simulink model "Experiment_2_cs"  (Simulink 8.4)
settings: Solver=ode5  SolverMode=SingleTasking  StartTime=0.0  StopTime=inf  FixedStep=1/100  RelTol=1e-3
PreLoadFcn:
  | mbxruntime.callbacks.PreLoadFcn(bdroot);
PostLoadFcn:
  | mbxruntime.callbacks.PostLoadFcn(bdroot);
InitFcn:
  | mbxruntime.callbacks.InitFcn(bdroot);
StartFcn:
  | mbxruntime.callbacks.StartFcn(bdroot);
StopFcn:
  | mbxruntime.callbacks.StopFcn(bdroot);
undefined symbols (not defined in the file or in its folder): dfreq, gray, InitImageOutputDir, Rec, SDTV, strel, warningInitialVelocity, x0
libraries: simulink x43, PreScanSimulinkLibrary x19, visiontextngfix x15, simulink_extras x11, visionconversions x3, PreScanUsefulBlocks x3, visionsinks x2, visionstatistics x1, visionmorphops x1, visionanalysis x1
(part 5 of 8)

== system Experiment_2_cs/Audi_A8_1/ENABLED/Trajectories/TrajCoGOffset ==
  State In : Inport
  Add : Sum  Inputs=+-+
  Add1 : Sum
  ApplyRotation : PreScanSimulinkLibrary/ApplyRotation
  ApplyRotation1 : PreScanSimulinkLibrary/ApplyRotation
  CoG Offset : Constant  Value=[0 0 CoGOffsetZ]
  Degrees to Radians : simulink_extras/Transformations/Degrees to Radians
  Demux1 : Demux  Outputs=[3 3 3]
  Mux : Mux  Inputs=[3 3 3]
  Orientation : Constant  Value=[InitRoll InitPitch 0]
  State Out : Outport
  wires:
  State In/1 -> Demux1/1
  Demux1/1 -> Add/1
  Add/1 -> Mux/1
  Demux1/3 -> Mux/3, Add1/2
  Mux/1 -> State Out/1
  Demux1/2 -> Mux/2
  Orientation/1 -> Degrees to Radians/1
  ApplyRotation/1 -> Add/3
  ApplyRotation1/1 -> Add/2
  Add1/1 -> ApplyRotation/2
  CoG Offset/1 -> ApplyRotation1/1, ApplyRotation/1
  Degrees to Radians/1 -> Add1/1, ApplyRotation1/2

== system Experiment_2_cs/Audi_A8_1/ENABLED/Trajectories/Trajectory_2 ==
  From Workspace : FromWorkspace  VariableName=trajectory  SampleTime=TimeStep  OutputAfterFinalValue=Holding final value
  From Workspace1 : FromWorkspace  VariableName=trajectory  SampleTime=TimeStep  OutputAfterFinalValue=Setting to zero
  Mux : Mux  Inputs=2
  Selector1 : Selector  InputPortWidth=24  Indices=[7:18]
  Selector9 : Selector  InputPortWidth=24  Indices=[1:6]
  trajectory : Outport
  wires:
  From Workspace/1 -> Selector9/1
  From Workspace1/1 -> Selector1/1
  Mux/1 -> trajectory/1
  Selector9/1 -> Mux/1
  Selector1/1 -> Mux/2

== system Experiment_2_cs/Audi_A8_1/ENABLED/V2X_210_Generic_Filter/Filter ==
  In : Inport
  Filter : MATLAB Function  TreatAsAtomicUnit=on
  Zero : Constant  Value=0  OutDataTypeStr=Bus: PRESCAN_V2X_USER_GENERIC_MESSAGE
  Out : Outport
  wires:
  Zero/1 -> Filter/2(z)
  Filter/1(y) -> Out/1
  In/1 -> Filter/1(u)

== system Experiment_2_cs/BMW_Z3_1/ENABLED/SELF_Demux/compas converter ==
  rotz [rad] : Inport
  cart2compas : Subsystem
  rad2deg : Gain  Gain=180/pi
  heading [deg] : Outport
  wires:
  rad2deg/1 -> cart2compas/1(Angle [deg])
  rotz [rad]/1 -> rad2deg/1
  cart2compas/1(heading [deg]) -> heading [deg]/1

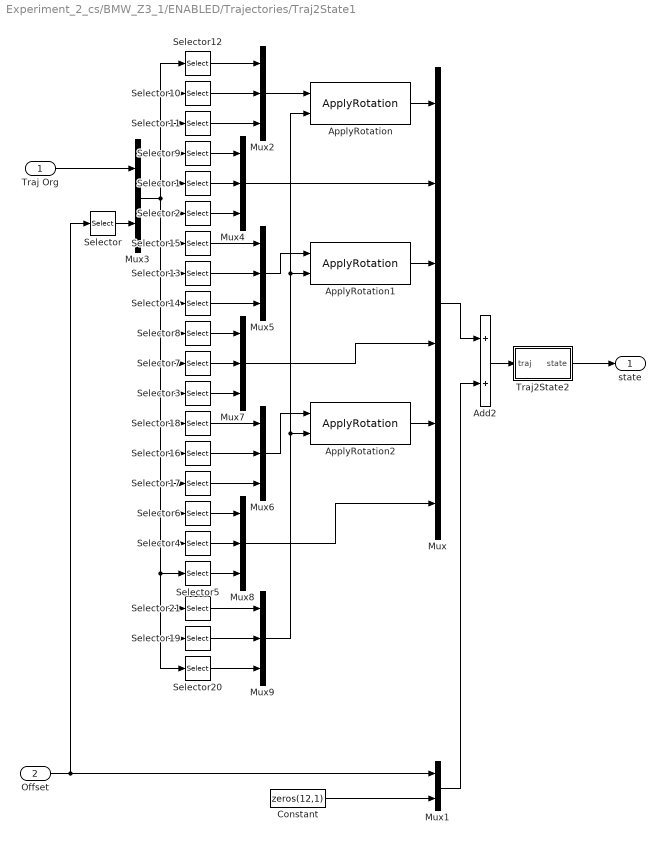
== system Experiment_2_cs/BMW_Z3_1/ENABLED/Trajectories/Traj2State1 ==
  Traj Org : Inport
  Offset : Inport  Port=2
  Add2 : Sum
  ApplyRotation : PreScanSimulinkLibrary/ApplyRotation
  ApplyRotation1 : PreScanSimulinkLibrary/ApplyRotation
  ApplyRotation2 : PreScanSimulinkLibrary/ApplyRotation
  Constant : Constant  Value=zeros(12,1)
  Mux : Mux  Inputs=6
  Mux1 : Mux  Inputs=2
  Mux{2,4..9} (7 alike) : Mux  Inputs=3
  Mux3 : Mux  Inputs=2
  Selector : Selector  InputPortWidth=6  Indices=[4 5 6]
  Selector1 : Selector  InputPortWidth=21  Indices=[5]
  Selector10 : Selector  InputPortWidth=21  Indices=[2]
  Selector11 : Selector  InputPortWidth=21  Indices=[3]
  Selector12 : Selector  InputPortWidth=21  Indices=[1]
  Selector13 : Selector  InputPortWidth=21  Indices=[8]
  Selector14 : Selector  InputPortWidth=21  Indices=[9]
  Selector15 : Selector  InputPortWidth=21  Indices=[7]
  Selector16 : Selector  InputPortWidth=21  Indices=[14]
  Selector17 : Selector  InputPortWidth=21  Indices=[15]
  Selector18 : Selector  InputPortWidth=21  Indices=[13]
  Selector19 : Selector  InputPortWidth=21  Indices=[20]
  Selector2 : Selector  InputPortWidth=21  Indices=[6]
  Selector20 : Selector  InputPortWidth=21  Indices=[21]
  Selector21 : Selector  InputPortWidth=21  Indices=[19]
  Selector3 : Selector  InputPortWidth=21  Indices=[12]
  Selector4 : Selector  InputPortWidth=21  Indices=[17]
  Selector5 : Selector  InputPortWidth=21  Indices=[18]
  Selector6 : Selector  InputPortWidth=21  Indices=[16]
  Selector7 : Selector  InputPortWidth=21  Indices=[11]
  Selector8 : Selector  InputPortWidth=21  Indices=[10]
  Selector9 : Selector  InputPortWidth=21  Indices=[4]
  Traj2State2 : Subsystem
  state : Outport
  wires:
  Mux9/1 -> ApplyRotation2/2, ApplyRotation1/2, ApplyRotation/2
  Selector20/1 -> Mux9/3
  Selector19/1 -> Mux9/2
  Selector21/1 -> Mux9/1
  Selector5/1 -> Mux8/3
  Selector4/1 -> Mux8/2
  Selector6/1 -> Mux8/1
  Mux8/1 -> Mux/6
  Mux6/1 -> ApplyRotation2/1
  Mux7/1 -> Mux/4
  ApplyRotation2/1 -> Mux/5
  Selector3/1 -> Mux7/3
  Selector7/1 -> Mux7/2
  Selector8/1 -> Mux7/1
  Mux4/1 -> Mux/2
  Mux5/1 -> ApplyRotation1/1
  ApplyRotation1/1 -> Mux/3
  Mux2/1 -> ApplyRotation/1
  ApplyRotation/1 -> Mux/1
  Selector2/1 -> Mux4/3
  Selector1/1 -> Mux4/2
  Selector9/1 -> Mux4/1
  Selector17/1 -> Mux6/3
  Selector16/1 -> Mux6/2
  Selector18/1 -> Mux6/1
  Selector14/1 -> Mux5/3
  Selector13/1 -> Mux5/2
  Selector15/1 -> Mux5/1
  Selector11/1 -> Mux2/3
  Selector10/1 -> Mux2/2
  Selector12/1 -> Mux2/1
  Mux3/1 -> Selector8/1, Selector7/1, Selector3/1, Selector18/1, Selector16/1, Selector17/1, Selector6/1, Selector20/1, Selector19/1, Selector21/1, Selector5/1, Selector4/1, Selector14/1, Selector13/1, Selector15/1, Selector2/1, Selector1/1, Selector9/1, Selector12/1, Selector10/1, Selector11/1
  Mux1/1 -> Add2/2
  Constant/1 -> Mux1/2
  Add2/1 -> Traj2State2/1(traj)
  Selector/1 -> Mux3/2
  Traj Org/1 -> Mux3/1
  Offset/1 -> Mux1/1, Selector/1
  Mux/1 -> Add2/1
  Traj2State2/1(state) -> state/1

== system Experiment_2_cs/BMW_Z3_1/ENABLED/Trajectories/TrajCoGOffset ==
  State In : Inport
  Add : Sum  Inputs=+-+
  Add1 : Sum
  ApplyRotation : PreScanSimulinkLibrary/ApplyRotation
  ApplyRotation1 : PreScanSimulinkLibrary/ApplyRotation
  CoG Offset : Constant  Value=[0 0 CoGOffsetZ]
  Degrees to Radians : simulink_extras/Transformations/Degrees to Radians
  Demux1 : Demux  Outputs=[3 3 3]
  Mux : Mux  Inputs=[3 3 3]
  Orientation : Constant  Value=[InitRoll InitPitch 0]
  State Out : Outport
  wires:
  State In/1 -> Demux1/1
  Demux1/1 -> Add/1
  Add/1 -> Mux/1
  Demux1/3 -> Mux/3, Add1/2
  Mux/1 -> State Out/1
  Demux1/2 -> Mux/2
  Orientation/1 -> Degrees to Radians/1
  ApplyRotation/1 -> Add/3
  ApplyRotation1/1 -> Add/2
  Add1/1 -> ApplyRotation/2
  CoG Offset/1 -> ApplyRotation1/1, ApplyRotation/1
  Degrees to Radians/1 -> Add1/1, ApplyRotation1/2

== system Experiment_2_cs/BMW_Z3_1/ENABLED/Trajectories/Trajectory_3 ==
  From Workspace : FromWorkspace  VariableName=trajectory  SampleTime=TimeStep  OutputAfterFinalValue=Holding final value
  From Workspace1 : FromWorkspace  VariableName=trajectory  SampleTime=TimeStep  OutputAfterFinalValue=Setting to zero
  Mux : Mux  Inputs=2
  Selector1 : Selector  InputPortWidth=24  Indices=[7:18]
  Selector9 : Selector  InputPortWidth=24  Indices=[1:6]
  trajectory : Outport
  wires:
  From Workspace/1 -> Selector9/1
  From Workspace1/1 -> Selector1/1
  Mux/1 -> trajectory/1
  Selector9/1 -> Mux/1
  Selector1/1 -> Mux/2

== system Experiment_2_cs/BMW_Z3_1/ENABLED/V2X_211_Generic_Filter/Filter ==
  In : Inport
  Filter : MATLAB Function  TreatAsAtomicUnit=on
  Zero : Constant  Value=0  OutDataTypeStr=Bus: PRESCAN_V2X_USER_GENERIC_MESSAGE
  Out : Outport
  wires:
  Zero/1 -> Filter/2(z)
  Filter/1(y) -> Out/1
  In/1 -> Filter/1(u)

== system Experiment_2_cs/CollisionDetection/DISABLED/GND1/GND_DATA ==
  GND_ObjectID1 : Constant  Value=uint32(0)
  GND_ObjectID2 : Constant  Value=uint32(0)
  buscreator : BusCreator  Inputs=2  OutDataTypeStr=Bus: PRESCAN_COLLISIONDETECTION_DATA  NonVirtualBus=on
  bus : Outport  OutDataTypeStr=Bus: PRESCAN_COLLISIONDETECTION_DATA
  wires:
  GND_ObjectID1/1 -> buscreator/1  "ObjectID1"
  GND_ObjectID2/1 -> buscreator/2  "ObjectID2"
  buscreator/1 -> bus/1

== system Experiment_2_cs/CollisionDetection/DISABLED/GND1/GND_HEADER ==
  GND_valid : Constant  Value=boolean(0)
  buscreator : BusCreator  Inputs=1  OutDataTypeStr=Bus: PRESCAN_HEADER  NonVirtualBus=on
  bus : Outport  OutDataTypeStr=Bus: PRESCAN_HEADER
  wires:
  GND_valid/1 -> buscreator/1  "valid"
  buscreator/1 -> bus/1

== system Experiment_2_cs/Male_RegularAni_1/ENABLED/Animation/animation mode ==
  vel : Inport
  Data Type Conversion : DataTypeConversion  OutDataTypeStr=double
  Fcn : Fcn  Expr=sqrt(u(1)^2+u(2)^2+u(3)^2)
  Running : simulink/Logic and Bit Operations/Compare To Constant  relop=>=  const=MWS  OutDataTypeStr=uint8  ZeroCross=off
  Sum : Sum  Inputs=|++
  Walking : simulink/Logic and Bit Operations/Compare To Zero  relop=~=  OutDataTypeStr=uint8  ZeroCross=off
  mode : Outport
  wires:
  vel/1 -> Fcn/1
  Sum/1 -> Data Type Conversion/1
  Walking/1 -> Sum/1
  Running/1 -> Sum/2
  Fcn/1 -> Walking/1, Running/1
  Data Type Conversion/1 -> mode/1

== system Experiment_2_cs/Male_RegularAni_1/ENABLED/Animation/elapsed track ==
  vel : Inport
  Discrete-Time Integrator : DiscreteIntegrator  SampleTime=-1
  Fcn : Fcn  Expr=sqrt(u(1)^2 + u(2)^2 + u(3)^2)
  s : Outport
  wires:
  Fcn/1 -> Discrete-Time Integrator/1
  vel/1 -> Fcn/1
  Discrete-Time Integrator/1 -> s/1

== system Experiment_2_cs/Male_RegularAni_1/ENABLED/SELF_Demux/compas converter ==
  rotz [rad] : Inport
  cart2compas : Subsystem
  rad2deg : Gain  Gain=180/pi
  heading [deg] : Outport
  wires:
  rad2deg/1 -> cart2compas/1(Angle [deg])
  rotz [rad]/1 -> rad2deg/1
  cart2compas/1(heading [deg]) -> heading [deg]/1

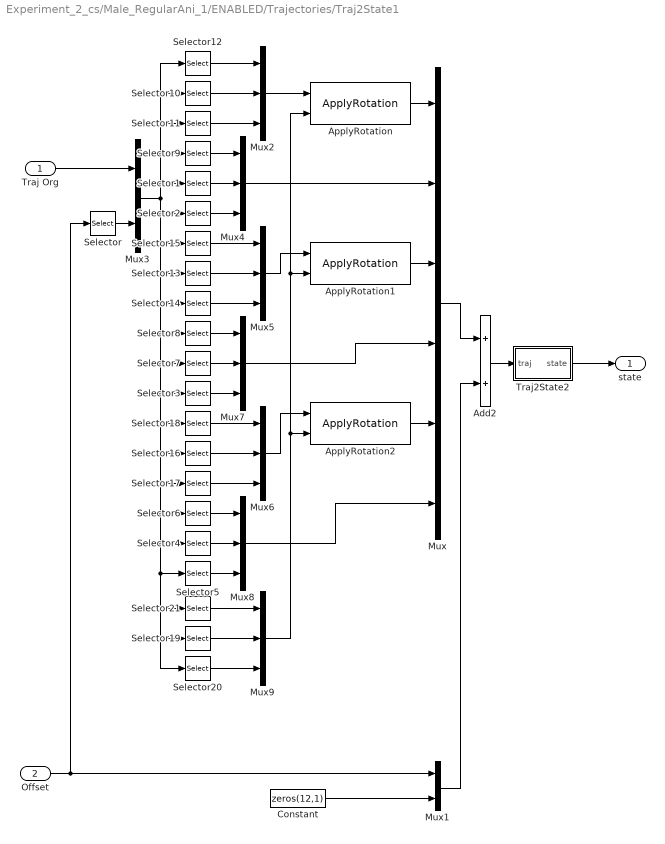
== system Experiment_2_cs/Male_RegularAni_1/ENABLED/Trajectories/Traj2State1 ==
  Traj Org : Inport
  Offset : Inport  Port=2
  Add2 : Sum
  ApplyRotation : PreScanSimulinkLibrary/ApplyRotation
  ApplyRotation1 : PreScanSimulinkLibrary/ApplyRotation
  ApplyRotation2 : PreScanSimulinkLibrary/ApplyRotation
  Constant : Constant  Value=zeros(12,1)
  Mux : Mux  Inputs=6
  Mux1 : Mux  Inputs=2
  Mux{2,4..9} (7 alike) : Mux  Inputs=3
  Mux3 : Mux  Inputs=2
  Selector : Selector  InputPortWidth=6  Indices=[4 5 6]
  Selector1 : Selector  InputPortWidth=21  Indices=[5]
  Selector10 : Selector  InputPortWidth=21  Indices=[2]
  Selector11 : Selector  InputPortWidth=21  Indices=[3]
  Selector12 : Selector  InputPortWidth=21  Indices=[1]
  Selector13 : Selector  InputPortWidth=21  Indices=[8]
  Selector14 : Selector  InputPortWidth=21  Indices=[9]
  Selector15 : Selector  InputPortWidth=21  Indices=[7]
  Selector16 : Selector  InputPortWidth=21  Indices=[14]
  Selector17 : Selector  InputPortWidth=21  Indices=[15]
  Selector18 : Selector  InputPortWidth=21  Indices=[13]
  Selector19 : Selector  InputPortWidth=21  Indices=[20]
  Selector2 : Selector  InputPortWidth=21  Indices=[6]
  Selector20 : Selector  InputPortWidth=21  Indices=[21]
  Selector21 : Selector  InputPortWidth=21  Indices=[19]
  Selector3 : Selector  InputPortWidth=21  Indices=[12]
  Selector4 : Selector  InputPortWidth=21  Indices=[17]
  Selector5 : Selector  InputPortWidth=21  Indices=[18]
  Selector6 : Selector  InputPortWidth=21  Indices=[16]
  Selector7 : Selector  InputPortWidth=21  Indices=[11]
  Selector8 : Selector  InputPortWidth=21  Indices=[10]
  Selector9 : Selector  InputPortWidth=21  Indices=[4]
  Traj2State2 : Subsystem
  state : Outport
  wires:
  Mux9/1 -> ApplyRotation2/2, ApplyRotation1/2, ApplyRotation/2
  Selector20/1 -> Mux9/3
  Selector19/1 -> Mux9/2
  Selector21/1 -> Mux9/1
  Selector5/1 -> Mux8/3
  Selector4/1 -> Mux8/2
  Selector6/1 -> Mux8/1
  Mux8/1 -> Mux/6
  Mux6/1 -> ApplyRotation2/1
  Mux7/1 -> Mux/4
  ApplyRotation2/1 -> Mux/5
  Selector3/1 -> Mux7/3
  Selector7/1 -> Mux7/2
  Selector8/1 -> Mux7/1
  Mux4/1 -> Mux/2
  Mux5/1 -> ApplyRotation1/1
  ApplyRotation1/1 -> Mux/3
  Mux2/1 -> ApplyRotation/1
  ApplyRotation/1 -> Mux/1
  Selector2/1 -> Mux4/3
  Selector1/1 -> Mux4/2
  Selector9/1 -> Mux4/1
  Selector17/1 -> Mux6/3
  Selector16/1 -> Mux6/2
  Selector18/1 -> Mux6/1
  Selector14/1 -> Mux5/3
  Selector13/1 -> Mux5/2
  Selector15/1 -> Mux5/1
  Selector11/1 -> Mux2/3
  Selector10/1 -> Mux2/2
  Selector12/1 -> Mux2/1
  Mux3/1 -> Selector8/1, Selector7/1, Selector3/1, Selector18/1, Selector16/1, Selector17/1, Selector6/1, Selector20/1, Selector19/1, Selector21/1, Selector5/1, Selector4/1, Selector14/1, Selector13/1, Selector15/1, Selector2/1, Selector1/1, Selector9/1, Selector12/1, Selector10/1, Selector11/1
  Mux1/1 -> Add2/2
  Constant/1 -> Mux1/2
  Add2/1 -> Traj2State2/1(traj)
  Selector/1 -> Mux3/2
  Traj Org/1 -> Mux3/1
  Offset/1 -> Mux1/1, Selector/1
  Mux/1 -> Add2/1
  Traj2State2/1(state) -> state/1

== system Experiment_2_cs/Male_RegularAni_1/ENABLED/Trajectories/TrajCoGOffset ==
  State In : Inport
  Add : Sum  Inputs=+-+
  Add1 : Sum
  ApplyRotation : PreScanSimulinkLibrary/ApplyRotation
  ApplyRotation1 : PreScanSimulinkLibrary/ApplyRotation
  CoG Offset : Constant  Value=[0 0 CoGOffsetZ]
  Degrees to Radians : simulink_extras/Transformations/Degrees to Radians
  Demux1 : Demux  Outputs=[3 3 3]
  Mux : Mux  Inputs=[3 3 3]
  Orientation : Constant  Value=[InitRoll InitPitch 0]
  State Out : Outport
  wires:
  State In/1 -> Demux1/1
  Demux1/1 -> Add/1
  Add/1 -> Mux/1
  Demux1/3 -> Mux/3, Add1/2
  Mux/1 -> State Out/1
  Demux1/2 -> Mux/2
  Orientation/1 -> Degrees to Radians/1
  ApplyRotation/1 -> Add/3
  ApplyRotation1/1 -> Add/2
  Add1/1 -> ApplyRotation/2
  CoG Offset/1 -> ApplyRotation1/1, ApplyRotation/1
  Degrees to Radians/1 -> Add1/1, ApplyRotation1/2

== system Experiment_2_cs/Male_RegularAni_1/ENABLED/Trajectories/Trajectory_1 ==
  From Workspace : FromWorkspace  VariableName=trajectory  SampleTime=TimeStep  OutputAfterFinalValue=Holding final value
  From Workspace1 : FromWorkspace  VariableName=trajectory  SampleTime=TimeStep  OutputAfterFinalValue=Setting to zero
  Mux : Mux  Inputs=2
  Selector1 : Selector  InputPortWidth=24  Indices=[7:18]
  Selector9 : Selector  InputPortWidth=24  Indices=[1:6]
  trajectory : Outport
  wires:
  From Workspace/1 -> Selector9/1
  From Workspace1/1 -> Selector1/1
  Mux/1 -> trajectory/1
  Selector9/1 -> Mux/1
  Selector1/1 -> Mux/2

== system Experiment_2_cs/TIS_1/DISABLED/GND1/GND_DATA ==
  GND_ActiveBeamID : Constant  Value=uint32(0)
  GND_Alpha : Constant  Value=0
  GND_Beta : Constant  Value=0
  GND_DopplerVelocity : Constant  Value=0
  GND_DopplerVelocityRotationX : Constant  Value=0
  GND_DopplerVelocityRotationY : Constant  Value=0
  GND_DopplerVelocityRotationZ : Constant  Value=0
  GND_DopplerVelocityTranslationX : Constant  Value=0
  GND_DopplerVelocityTranslationY : Constant  Value=0
  GND_DopplerVelocityTranslationZ : Constant  Value=0
  GND_EnergyLoss : Constant  Value=0
  GND_Phi : Constant  Value=0
  GND_Range : Constant  Value=0
  GND_TargetID : Constant  Value=uint32(0)
  GND_TargetTypeID : Constant  Value=uint32(0)
  GND_Theta : Constant  Value=0
  buscreator : BusCreator  Inputs=16  OutDataTypeStr=Bus: PRESCAN_SCANNERSENSOR_DATA  NonVirtualBus=on
  bus : Outport  OutDataTypeStr=Bus: PRESCAN_SCANNERSENSOR_DATA
  wires:
  GND_ActiveBeamID/1 -> buscreator/1  "ActiveBeamID"
  GND_Range/1 -> buscreator/2  "Range"
  GND_DopplerVelocity/1 -> buscreator/3  "DopplerVelocity"
  GND_Theta/1 -> buscreator/4  "Theta"
  GND_Phi/1 -> buscreator/5  "Phi"
  GND_TargetID/1 -> buscreator/6  "TargetID"
  GND_TargetTypeID/1 -> buscreator/7  "TargetTypeID"
  GND_EnergyLoss/1 -> buscreator/8  "EnergyLoss"
  GND_Alpha/1 -> buscreator/9  "Alpha"
  GND_Beta/1 -> buscreator/10  "Beta"
  GND_DopplerVelocityTranslationX/1 -> buscreator/11  "DopplerVelocityTranslationX"
  GND_DopplerVelocityTranslationY/1 -> buscreator/12  "DopplerVelocityTranslationY"
  GND_DopplerVelocityTranslationZ/1 -> buscreator/13  "DopplerVelocityTranslationZ"
  GND_DopplerVelocityRotationX/1 -> buscreator/14  "DopplerVelocityRotationX"
  GND_DopplerVelocityRotationY/1 -> buscreator/15  "DopplerVelocityRotationY"
  GND_DopplerVelocityRotationZ/1 -> buscreator/16  "DopplerVelocityRotationZ"
  buscreator/1 -> bus/1

== system Experiment_2_cs/TIS_1/DISABLED/GND1/GND_HEADER ==
  GND_valid : Constant  Value=boolean(0)
  buscreator : BusCreator  Inputs=1  OutDataTypeStr=Bus: PRESCAN_HEADER  NonVirtualBus=on
  bus : Outport  OutDataTypeStr=Bus: PRESCAN_HEADER
  wires:
  GND_valid/1 -> buscreator/1  "valid"
  buscreator/1 -> bus/1

== system Experiment_2_cs/TIS_2/DISABLED/GND1/GND_DATA ==
  GND_ActiveBeamID : Constant  Value=uint32(0)
  GND_Alpha : Constant  Value=0
  GND_Beta : Constant  Value=0
  GND_DopplerVelocity : Constant  Value=0
  GND_DopplerVelocityRotationX : Constant  Value=0
  GND_DopplerVelocityRotationY : Constant  Value=0
  GND_DopplerVelocityRotationZ : Constant  Value=0
  GND_DopplerVelocityTranslationX : Constant  Value=0
  GND_DopplerVelocityTranslationY : Constant  Value=0
  GND_DopplerVelocityTranslationZ : Constant  Value=0
  GND_EnergyLoss : Constant  Value=0
  GND_Phi : Constant  Value=0
  GND_Range : Constant  Value=0
  GND_TargetID : Constant  Value=uint32(0)
  GND_TargetTypeID : Constant  Value=uint32(0)
  GND_Theta : Constant  Value=0
  buscreator : BusCreator  Inputs=16  OutDataTypeStr=Bus: PRESCAN_SCANNERSENSOR_DATA  NonVirtualBus=on
  bus : Outport  OutDataTypeStr=Bus: PRESCAN_SCANNERSENSOR_DATA
  wires:
  GND_ActiveBeamID/1 -> buscreator/1  "ActiveBeamID"
  GND_Range/1 -> buscreator/2  "Range"
  GND_DopplerVelocity/1 -> buscreator/3  "DopplerVelocity"
  GND_Theta/1 -> buscreator/4  "Theta"
  GND_Phi/1 -> buscreator/5  "Phi"
  GND_TargetID/1 -> buscreator/6  "TargetID"
  GND_TargetTypeID/1 -> buscreator/7  "TargetTypeID"
  GND_EnergyLoss/1 -> buscreator/8  "EnergyLoss"
  GND_Alpha/1 -> buscreator/9  "Alpha"
  GND_Beta/1 -> buscreator/10  "Beta"
  GND_DopplerVelocityTranslationX/1 -> buscreator/11  "DopplerVelocityTranslationX"
  GND_DopplerVelocityTranslationY/1 -> buscreator/12  "DopplerVelocityTranslationY"
  GND_DopplerVelocityTranslationZ/1 -> buscreator/13  "DopplerVelocityTranslationZ"
  GND_DopplerVelocityRotationX/1 -> buscreator/14  "DopplerVelocityRotationX"
  GND_DopplerVelocityRotationY/1 -> buscreator/15  "DopplerVelocityRotationY"
  GND_DopplerVelocityRotationZ/1 -> buscreator/16  "DopplerVelocityRotationZ"
  buscreator/1 -> bus/1

== system Experiment_2_cs/TIS_2/DISABLED/GND1/GND_HEADER ==
  GND_valid : Constant  Value=boolean(0)
  buscreator : BusCreator  Inputs=1  OutDataTypeStr=Bus: PRESCAN_HEADER  NonVirtualBus=on
  bus : Outport  OutDataTypeStr=Bus: PRESCAN_HEADER
  wires:
  GND_valid/1 -> buscreator/1  "valid"
  buscreator/1 -> bus/1

== system Experiment_2_cs/Audi_A8_1/ENABLED/Dynamics_Simple/Chassis/Bicycle_model_[XYZ] ==
  DeltaWheel_[rad] : Inport
  zFront_[m]_dzFront_[ms-1] : Inport  Port=2  PortDimensions=2
  zRear_[m]_dzRear_[ms-1] : Inport  Port=3  PortDimensions=2
  BrakePressure_[bar] : Inport  Port=4
  DriveTorque_[Nm] : Inport  Port=5
  v0_[ms-1] : Inport  Port=6
  |vx|_[ms-1] : Inport  Port=7
  Fy_rear_[N] : Inport  Port=8
  Fy_front_[N] : Inport  Port=9
  Demux : Demux  Outputs=2
  Demux1 : Demux  Outputs=2
  Fyi --> Fy / Mz : Subsystem
  X_Motion : Subsystem
  Y & Yaw_Motion : Subsystem
  "Z, Pitch_Motion & Roll_Motion" : Subsystem
  |vx|_[ms-1]1 : Outport
  vy_[ms-1] : Outport  Port=2
  vz_[ms-1] : Outport  Port=3
  RollAngle_[rad] : Outport  Port=4
  RollRate_[rads-1] : Outport  Port=5
  YawAngle_[rads-1] : Outport  Port=6
  Vx_[ms-1] : Outport  Port=7
  PitchAngle_[rad] : Outport  Port=8
  YawAngle_[rad] : Outport  Port=9
  ax_[ms-2] : Outport  Port=10
  ay_[ms-2] : Outport  Port=11
  wires:
  Fyi --> Fy / Mz/1(Fy_[N]) -> Y & Yaw_Motion/2(Fy_[N])  "Fy_[N]"
  Fyi --> Fy / Mz/2(Mz_[Nm]) -> Y & Yaw_Motion/3(Mz_[Nm])  "Mz_[Nm]"
  Y & Yaw_Motion/1(|vx|_[ms-1]1) -> |vx|_[ms-1]1/1  "|vx|_[ms-1]"
  Y & Yaw_Motion/2(vy_[ms-1]) -> vy_[ms-1]/1  "vy_[ms-1]"
  Y & Yaw_Motion/5(YawAngle_[rad]) -> YawAngle_[rad]/1  "YawAngle_[rad]"
  v0_[ms-1]/1 -> X_Motion/3(v0_[ms-1])  "v0_[ms-1]"
  BrakePressure_[bar]/1 -> X_Motion/2(BrakePressure_[bar])  "BrakePressure_[bar]"
  DriveTorque_[Nm]/1 -> X_Motion/1(DriveTorque_[Nm])  "DriveTorque_[Nm]"
  X_Motion/2(ax_[ms-2]) -> ax_[ms-2]/1, [ax]  "ax_[ms-2]"
  X_Motion/1(vx_[ms-1]) -> Vx_[ms-1]/1, [vx]  "vx_[ms-1]"
  [ax] -> "Z, Pitch_Motion & Roll_Motion"/3(ax)
  Demux/1 -> "Z, Pitch_Motion & Roll_Motion"/5(zFront_[m])
  Demux/2 -> "Z, Pitch_Motion & Roll_Motion"/6(dzFront_[ms-1])
  Demux1/1 -> "Z, Pitch_Motion & Roll_Motion"/7(zRear_[m])
  Demux1/2 -> "Z, Pitch_Motion & Roll_Motion"/8(dzRear_[ms-1])
  zRear_[m]_dzRear_[ms-1]/1 -> Demux1/1
  zFront_[m]_dzFront_[ms-1]/1 -> Demux/1
  "Z, Pitch_Motion & Roll_Motion"/2(vz_[ms-1]) -> vz_[ms-1]/1  "vz_[ms-1]"
  DeltaWheel_[rad]/1 -> Fyi --> Fy / Mz/1(DeltaWheel_[rad])
  Fy_front_[N]/1 -> Fyi --> Fy / Mz/2(Fy_f_[N])
  Fy_rear_[N]/1 -> Fyi --> Fy / Mz/3(Fy_r_[N])
  |vx|_[ms-1]/1 -> Y & Yaw_Motion/1(|vx|_[ms-1])
  Y & Yaw_Motion/3(ay_[ms-2]) -> [ay], ay_[ms-2]/1  "ay_[ms-2]"
  [ay] -> "Z, Pitch_Motion & Roll_Motion"/4(ay)
  "Z, Pitch_Motion & Roll_Motion"/3(RollAngle_[rad]) -> RollAngle_[rad]/1  "RollAngle_[rad]"
  "Z, Pitch_Motion & Roll_Motion"/4(RollRate_[rads-1]) -> RollRate_[rads-1]/1  "RollRate_[rads-1]"
  [dYaw] -> "Z, Pitch_Motion & Roll_Motion"/2(dYaw)
  [vx] -> "Z, Pitch_Motion & Roll_Motion"/1(vx)
  Y & Yaw_Motion/4(dYawAngle_[rads-1]) -> YawAngle_[rads-1]/1, [dYaw]  "dYawAngle_[rads-1]"
  "Z, Pitch_Motion & Roll_Motion"/1(pitchAngle_[rad]) -> PitchAngle_[rad]/1  "PitchAngle_[rad]"

== system Experiment_2_cs/Audi_A8_1/ENABLED/Dynamics_Simple/Chassis/FrontTyre ==
  note: alpha limiter
      | [-1 ... 1]
  note: relax_on
      | ON: 1
      | OFF: 0
  note: MOTORCYCLE ONLY
  note: VEHICLE + MOTORCYCLE
  DeltaWheel_[rad] : Inport
  |vx|_[ms-1] : Inport  Port=2
  vy_[ms-1] : Inport  Port=3
  dYawAngle_[rads-1] : Inport  Port=4
  RollAngle_[rad] : Inport  Port=5
  AlphaFront : Subsystem
  Compare To Zero : simulink/Logic and Bit Operations/Compare To Zero  relop===  OutDataTypeStr=boolean  ZeroCross=off
  Configurable Subsystem : Subsystem  BlockChoice=Integrator  mask{ComputationMode=ComputationMode}
      mask prompts: ComputationMode "Computation mode:"
      mask init:
      | SetComputationMode(gcb,ComputationMode);
      settings: AttributesFormatString=%<BlockChoice>  OpenFcn=BringToFront(gcb);  MemberBlocks=Discrete-Time Integrator,Integrator
      settings: TemplateBlock=|
      | PreScanSimulinkLibrary/Configurable Subsystems/integral with reset and limits
      | for slip angle/Configurable
      | Subsystem
  Configurable Subsystem1 : Subsystem  BlockChoice=Integrator  mask{ComputationMode=ComputationMode}
      mask prompts: ComputationMode "Computation mode:"
      mask init:
      | SetComputationMode(gcb,ComputationMode);
      settings: AttributesFormatString=%<BlockChoice>  OpenFcn=BringToFront(gcb);  MemberBlocks=Discrete-Time Integrator,Integrator
      settings: TemplateBlock=|
      | PreScanSimulinkLibrary/Configurable Subsystems/integral with reset/Configurable
      | Subsystem
  Constant : Constant  Value=p.relax_on
  Constant1 : Constant  Value=p.relax_on
  Constant2 : Constant  Value=p.VehMCSwitch
  Data Type Conversion : DataTypeConversion  OutDataTypeStr=double
  If MC : simulink/Logic and Bit Operations/Compare To Constant  relop===  const=2  OutDataTypeStr=uint8  ZeroCross=off
  K_gamma_front : Gain  Gain=p.Kgfront
  Linl : Fcn  Expr=(u(4) - u(5))/p.sigma_front*u(1)
  Linl1 : Fcn  Expr=(u(4) - u(5))/p.sigma_front*u(1)
  Mux1 : Mux  Inputs=3
  Mux2 : Mux  Inputs={3,1,1}
  Mux3 : Mux  Inputs={3,1,1}
  Prevent_instability_at_low_Vx : Subsystem
  Product : Product  RndMeth=Zero
  Sum : Sum  Inputs=|++  SaturateOnIntegerOverflow=on  InputSameDT=on  OutDataTypeStr=Inherit: Same as first input
  Sum1 : Sum  Inputs=|++
  Switch : Switch  Threshold=0.5  SaturateOnIntegerOverflow=on  InputSameDT=on
  Switch1 : Switch  Threshold=0.5  SaturateOnIntegerOverflow=on  InputSameDT=on
  alg.loop : Memory
  due to sign convention : Gain  Gain=-1  SaturateOnIntegerOverflow=on  OutDataTypeStr=Inherit: Same as input  ParamDataTypeStr=Inherit: Same as input
  front_tyre : Gain  Gain=p.Kfront
  FyFront_[N] : Outport
  wires:
  Prevent_instability_at_low_Vx/1(alpha [rad]) -> Mux2/2, Switch/3
  Sum/1 -> Prevent_instability_at_low_Vx/1(alpha[rad])  "AlphaStatFront_[rad]"
  Switch/1 -> front_tyre/1  "AlphaFront_[rad]"
  Constant/1 -> Switch/2
  Sum1/1 -> FyFront_[N]/1  "FyFront_[N]"
  Mux2/1 -> Linl/1
  Linl/1 -> Configurable Subsystem/1(In1)
  Configurable Subsystem/1(Out1) -> Mux2/3, Switch/1  "AlphaRelaxFront_[rad]"
  AlphaFront/1(Alpha) -> Sum/1
  Mux1/1 -> Prevent_instability_at_low_Vx/2(In), AlphaFront/1(In), Mux2/1, Mux3/1
  |vx|_[ms-1]/1 -> Mux1/1, Compare To Zero/1
  vy_[ms-1]/1 -> Mux1/2
  dYawAngle_[rads-1]/1 -> Mux1/3
  alg.loop/1 -> Switch1/3
  Configurable Subsystem1/1(Out1) -> Mux3/3, Switch1/1  "GammaRelaxFront_[rad]"
  Linl1/1 -> Configurable Subsystem1/1(In1)
  Mux3/1 -> Linl1/1
  Constant1/1 -> Switch1/2
  due to sign convention/1 -> alg.loop/1, Mux3/2  "GammaStatFront_[rad]"
  RollAngle_[rad]/1 -> due to sign convention/1
  front_tyre/1 -> Sum1/1
  Constant2/1 -> If MC/1
  If MC/1 -> Data Type Conversion/1
  K_gamma_front/1 -> Product/1
  Product/1 -> Sum1/2
  Data Type Conversion/1 -> Product/2
  Compare To Zero/1 -> [reset]
  [reset] -> Configurable Subsystem/2(In2)
  [reset] -> Configurable Subsystem1/2(In2)
  DeltaWheel_[rad]/1 -> Sum/2  "DeltaWheel_[rad]"
  Switch1/1 -> K_gamma_front/1  "GammaFront_[rad]"

== system Experiment_2_cs/Audi_A8_1/ENABLED/Dynamics_Simple/Chassis/MuxDynState ==
  note: The position inputs are computed by the
      | integrated velocity.
  note: mode: Dynamics
      | VelVEHICLE
      | wrt VEH
  note: AnglesVEHICLE
      | wrtGLOB
  vx [ms-1] : Inport
  vy [ms-1] : Inport  Port=2
  vz [ms-1] : Inport  Port=3
  R [rad] : Inport  Port=4
  P [rad] : Inport  Port=5
  Y [rad] : Inport  Port=6
  Configurable Subsystem1 : Subsystem  BlockChoice=Integrator  mask{ComputationMode=ComputationMode}
      mask prompts: ComputationMode "Computation mode:"
      mask init:
      | SetComputationMode(gcb,ComputationMode);
      settings: AttributesFormatString=%<BlockChoice>  OpenFcn=BringToFront(gcb);  MemberBlocks=Discrete-Time Integrator,Integrator
      settings: TemplateBlock=|
      | PreScanSimulinkLibrary/Configurable Subsystems/integral/Configurable
      | Subsystem1
  Ground : Ground
  Ground1 : Ground
  Mux : Mux  Inputs=[3 3 3]
  Mux1 : Mux  Inputs=3
  Mux2 : Mux  Inputs=3
  Transformation_BODY2GLOBAL : Subsystem
  mux3 : Mux  Inputs=3
  State : Outport
  wires:
  Ground1/1 -> mux3/2  "pitch"
  Y [rad]/1 -> Mux2/3, mux3/3  "yaw"
  P [rad]/1 -> Mux2/2
  R [rad]/1 -> Mux2/1
  vz [ms-1]/1 -> Mux1/3
  vy [ms-1]/1 -> Mux1/2
  vx [ms-1]/1 -> Mux1/1
  Mux2/1 -> Mux/3
  Transformation_BODY2GLOBAL/1(Vvector_GLOBAL_[m/s]) -> Configurable Subsystem1/1(In1), Mux/2  "VelVEH wrt  GLOB"
  mux3/1 -> Transformation_BODY2GLOBAL/2(angles_BODYwrtGLOB_[rad])
  Ground/1 -> mux3/1  "roll"
  Mux/1 -> State/1
  Mux1/1 -> Transformation_BODY2GLOBAL/1(Vvector_BODY_[m/s])
  Configurable Subsystem1/1(Out1) -> Mux/1  "PosVEH wrt  GLOB"

== system Experiment_2_cs/Audi_A8_1/ENABLED/Dynamics_Simple/Chassis/Power Assisted Steering ==
  note: MOTORCYCLE
  note: VEHICLE
  note: Reverse steering direction for negative velocities
  Vx_[ms-1] : Inport
  Delta_in_[deg] : Inport  Port=2
  Constant : Constant
  Constant1 : Constant  Value=p.VehMCSwitch
  Lookup Table : Lookup  InputValues=[0 35 45 100]  Table=[1 1 0.2 0.2]
  Multiport Switch : MultiPortSwitch  Inputs=2
  Product : Product  Inputs=3  RndMeth=Zero
  Sign : Signum
  Delta_out_[deg] : Outport
  wires:
  Vx_[ms-1]/1 -> Lookup Table/1, Sign/1
  Delta_in_[deg]/1 -> Product/3
  Constant1/1 -> Multiport Switch/1
  Constant/1 -> Multiport Switch/3
  Lookup Table/1 -> Multiport Switch/2
  Multiport Switch/1 -> Product/2
  Product/1 -> Delta_out_[deg]/1
  Sign/1 -> Product/1

== system Experiment_2_cs/Audi_A8_1/ENABLED/Dynamics_Simple/Chassis/RearTyre ==
  note: alpha limiter
      | [-1 ... 1]
  note: relax_on
      | ON: 1
      | OFF: 0
  note: MOTORCYCLE ONLY
  note: VEHICLE + MOTORCYCLE
  |vx|_[ms-1] : Inport
  vy_[ms-1] : Inport  Port=2
  dpsi_[rads-1] : Inport  Port=3
  RollAngle_[rad] : Inport  Port=4
  AlphaRear : Subsystem
  Compare To Zero : simulink/Logic and Bit Operations/Compare To Zero  relop===  OutDataTypeStr=boolean  ZeroCross=off
  Configurable Subsystem : Subsystem  BlockChoice=Integrator  mask{ComputationMode=ComputationMode}
      mask prompts: ComputationMode "Computation mode:"
      mask init:
      | SetComputationMode(gcb,ComputationMode);
      settings: AttributesFormatString=%<BlockChoice>  OpenFcn=BringToFront(gcb);  MemberBlocks=Discrete-Time Integrator,Integrator
      settings: TemplateBlock=|
      | PreScanSimulinkLibrary/Configurable Subsystems/integral with reset/Configurable
      | Subsystem
  Configurable Subsystem1 : Subsystem  BlockChoice=Integrator  mask{ComputationMode=ComputationMode}
      mask prompts: ComputationMode "Computation mode:"
      mask init:
      | SetComputationMode(gcb,ComputationMode);
      settings: AttributesFormatString=%<BlockChoice>  OpenFcn=BringToFront(gcb);  MemberBlocks=Discrete-Time Integrator,Integrator
      settings: TemplateBlock=|
      | PreScanSimulinkLibrary/Configurable Subsystems/integral with reset and limits
      | for slip angle/Configurable
      | Subsystem
  Constant1 : Constant  Value=p.relax_on
  Constant2 : Constant  Value=p.relax_on
  Constant3 : Constant  Value=p.VehMCSwitch
  Data Type Conversion : DataTypeConversion  OutDataTypeStr=double
  If MC : simulink/Logic and Bit Operations/Compare To Constant  relop===  const=2  OutDataTypeStr=uint8  ZeroCross=off
  K_gamma_rear : Gain  Gain=p.Kgrear
  Linl : Fcn  Expr=(u(4) - u(5))/p.sigma_rear*u(1)
  Linl1 : Fcn  Expr=(u(4) - u(5))/p.sigma_rear*u(1)
  Mux1 : Mux  Inputs=3
  Mux2 : Mux  Inputs={3,1,1}
  Mux3 : Mux  Inputs={3,1,1}
  Prevent_instability_at_low_Vx : PreScanSimulinkLibrary/Simple_Vehicle_Dynamics/Chassis/FrontTyre/Prevent_instability_at_low_Vx
  Product : Product  RndMeth=Zero
  Sum1 : Sum  Inputs=|++
  Switch1 : Switch  Threshold=0.5  SaturateOnIntegerOverflow=on  InputSameDT=on
  Switch2 : Switch  Threshold=0.5  SaturateOnIntegerOverflow=on  InputSameDT=on
  alg.loop : Memory
  due to sign convention : Gain  Gain=-1  SaturateOnIntegerOverflow=on  OutDataTypeStr=Inherit: Same as input  ParamDataTypeStr=Inherit: Same as input
  rear_tyre : Gain  Gain=p.Krear
  FyRear_[N] : Outport
  wires:
  Prevent_instability_at_low_Vx/1 -> Switch1/3, Mux2/2
  AlphaRear/1(Alpha) -> Prevent_instability_at_low_Vx/1  "AlphaStatRear_[rad]"
  Switch1/1 -> rear_tyre/1  "AlphaRear_[rad]"
  Constant1/1 -> Switch1/2
  Sum1/1 -> FyRear_[N]/1  "FyRear_[N]"
  Mux2/1 -> Linl/1
  Linl/1 -> Configurable Subsystem1/1(In1)
  Configurable Subsystem1/1(Out1) -> Mux2/3, Switch1/1  "AlphaRelaxRear_[rad]"
  Mux1/1 -> Prevent_instability_at_low_Vx/2, AlphaRear/1(In), Mux2/1, Mux3/1
  |vx|_[ms-1]/1 -> Mux1/1, Compare To Zero/1
  vy_[ms-1]/1 -> Mux1/2
  dpsi_[rads-1]/1 -> Mux1/3
  alg.loop/1 -> Switch2/3
  Configurable Subsystem/1(Out1) -> Mux3/3, Switch2/1  "GammaRelaxRear_[rad]"
  Linl1/1 -> Configurable Subsystem/1(In1)
  Mux3/1 -> Linl1/1
  Constant2/1 -> Switch2/2
  due to sign convention/1 -> alg.loop/1, Mux3/2  "GammaStatRear_[rad]"
  RollAngle_[rad]/1 -> due to sign convention/1
  Constant3/1 -> If MC/1
  If MC/1 -> Data Type Conversion/1
  Product/1 -> Sum1/2
  Data Type Conversion/1 -> Product/2
  K_gamma_rear/1 -> Product/1
  rear_tyre/1 -> Sum1/1
  Compare To Zero/1 -> [reset]
  [reset] -> Configurable Subsystem1/2(In2)
  [reset] -> Configurable Subsystem/2(In2)
  Switch2/1 -> K_gamma_rear/1  "GammaFront_[rad]"

== system Experiment_2_cs/Audi_A8_1/ENABLED/Dynamics_Simple/Engine/Configurable Subsystem ==
  In1 : Inport
  Rate Limiter : TransferFcn  Denominator=[0.1 1]
  Out1 : Outport
  wires:
  In1/1 -> Rate Limiter/1
  Rate Limiter/1 -> Out1/1

== system Experiment_2_cs/Audi_A8_1/ENABLED/Dynamics_Simple/Engine/Configurable Subsystem1 ==
  In1 : Inport
  Integrator : Integrator  InitialCondition=p.rot_ini  LimitOutput=on  UpperSaturationLimit=p.rot_upp  LowerSaturationLimit=p.rot_low
  Out1 : Outport
  wires:
  In1/1 -> Integrator/1
  Integrator/1 -> Out1/1

== system Experiment_2_cs/Audi_A8_1/ENABLED/Dynamics_Simple/Gear: Auto Manual/If Action Subsystem ==
  In1 : Inport
  Action Port : ActionPort  PropagateVarSize=During execution  ActionType=then
  Out1 : Outport
  wires:
  In1/1 -> Out1/1

== system Experiment_2_cs/Audi_A8_1/ENABLED/Dynamics_Simple/Gear: Auto Manual/If Action Subsystem1 ==
  In1 : Inport
  Action Port : ActionPort  PropagateVarSize=During execution  ActionType=else
  Out1 : Outport
  wires:
  In1/1 -> Out1/1

== system Experiment_2_cs/Audi_A8_1/ENABLED/Dynamics_Simple/ShiftLogic/Detect Increase ==
  GearNr_[-] : Inport
  In2 : Inport  Port=2
  Constant : Constant
  Data Type Conversion : DataTypeConversion  OutDataTypeStr=double
  Data Type Conversion1 : DataTypeConversion  OutDataTypeStr=double
  Detect Increase : simulink/Logic and Bit Operations/Detect Increase  vinit=1  InputProcessing=Inherited  OutDataTypeStr=uint8
  If : If  NumInputs=2  IfExpression="u1==1 &  u2==1"
  If V0 higher of the from 2->3 shifting velocity : Subsystem  TreatAsAtomicUnit=on
  Merge : Merge
  Other : Subsystem  TreatAsAtomicUnit=on
  Out1 : Outport
  wires:
  If/2 -> Other/Action
  If V0 higher of the from 2->3 shifting velocity/1(Out1) -> Merge/1
  Other/1(Out1) -> Merge/2
  Detect Increase/1 -> Data Type Conversion/1
  Merge/1 -> Out1/1
  If/1 -> If V0 higher of the from 2->3 shifting velocity/Action
  Data Type Conversion1/1 -> If/2
  Data Type Conversion/1 -> If/1
  Constant/1 -> If V0 higher of the from 2->3 shifting velocity/1(In1)
  GearNr_[-]/1 -> Detect Increase/1
  In2/1 -> Data Type Conversion1/1, Other/1(In1)

== system Experiment_2_cs/Audi_A8_1/ENABLED/Dynamics_Simple/ShiftLogic/If Action Neutral ==
  In1 : Inport
  Action Port : ActionPort  InitializeStates=reset  PropagateVarSize=During execution  ActionType=then
  Out1 : Outport
  wires:
  In1/1 -> Out1/1

== system Experiment_2_cs/Audi_A8_1/ENABLED/Dynamics_Simple/ShiftLogic/If Action Normal ==
  In1 : Inport
  Action Port : ActionPort  InitializeStates=reset  PropagateVarSize=During execution  ActionType=else
  Out1 : Outport
  wires:
  In1/1 -> Out1/1

== system Experiment_2_cs/Audi_A8_1/ENABLED/Dynamics_Simple/ShiftLogic/If Action Reverse ==
  In1 : Inport
  Action Port : ActionPort  InitializeStates=reset  PropagateVarSize=During execution  ActionType=elseif
  Out1 : Outport
  wires:
  In1/1 -> Out1/1

== system Experiment_2_cs/Audi_A8_1/ENABLED/Dynamics_Simple/Transmission/Torque_Converter ==
  note: To compensate for no hydraulic connection when in neutral gear
  note: > 0
  note: <= 0
  nEngine_[rpm] : Inport
  nTransmission_[rpm] : Inport  Port=2
  Gear nr : Inport  Port=3
  Compare To Constant : simulink/Logic and Bit Operations/Compare To Constant  relop=<=  const=1  OutDataTypeStr=uint8  ZeroCross=off
  Compare To Zero : simulink/Logic and Bit Operations/Compare To Zero  relop=~=  OutDataTypeStr=uint8  ZeroCross=off
  Constant : Constant  Value=1/50
  Constant1 : Constant
  Constant2 : Constant
  Drag : Gain  Gain=-1
  FactorK : Lookup  InputValues=p.speedratio  Table=p.Kfactor*p.Kcorr  SaturateOnIntegerOverflow=on
  Impeller : Fcn  Expr=u^2
  Product : Product  RndMeth=Zero
  Product1 : Product  RndMeth=Zero
  Quotient : Product  Inputs=*/  SaturateOnIntegerOverflow=on  InputSameDT=on  OutDataTypeStr=Inherit: Same as first input
  SpeedRatio : Product  Inputs=*/  SaturateOnIntegerOverflow=on  InputSameDT=on  OutDataTypeStr=Inherit: Same as first input
  Sum : Sum  Inputs=|+-
  Switch : Switch  Criteria=u2 ~= 0  Threshold=0.5
  Switch1 : Switch  Criteria=u2 ~= 0
  TorqueRatio : Lookup  InputValues=[p.speedratio 1]  Table=[p.Torqueratio 0]  SaturateOnIntegerOverflow=on
  Turbine : Product  SaturateOnIntegerOverflow=on  InputSameDT=on  OutDataTypeStr=Inherit: Same as first input
  ImpellerTorque_[Nm] : Outport  InitialOutput=0
  TurbineTorque_[Nm] : Outport  Port=2  InitialOutput=0
  wires:
  nTransmission_[rpm]/1 -> SpeedRatio/1
  nEngine_[rpm]/1 -> Quotient/1, SpeedRatio/2
  Impeller/1 -> Product/2, Turbine/1
  SpeedRatio/1 -> FactorK/1, TorqueRatio/1, Compare To Constant/1, Sum/1
  FactorK/1 -> Quotient/2
  Quotient/1 -> Impeller/1
  Product/1 -> ImpellerTorque_[Nm]/1
  Switch/1 -> Product/1, Product1/1
  Constant/1 -> Switch/3
  Constant1/1 -> Switch/1
  Gear nr/1 -> Compare To Zero/1
  Compare To Zero/1 -> Switch/2
  Switch1/1 -> Product1/2
  Product1/1 -> TurbineTorque_[Nm]/1
  Drag/1 -> Switch1/3
  Sum/1 -> Drag/1
  Constant2/1 -> Sum/2
  Compare To Constant/1 -> Switch1/2
  TorqueRatio/1 -> Turbine/2
  Turbine/1 -> Switch1/1

== system Experiment_2_cs/Audi_A8_1/ENABLED/Dynamics_Simple/Transmission/Transmission_Ratio ==
  tTransmissionIn_[Nm] : Inport
  GearNr_[-] : Inport  Port=2
  nTransmissionOut_[rpm] : Inport  Port=3
  Ensure positive TransmissionRPM : Abs
  If : If  IfExpression=u1 == 0  ElseIfExpressions=u1 == -1
  If Action Neutral : Subsystem  TreatAsAtomicUnit=on
  If Action Normal : Subsystem  TreatAsAtomicUnit=on
  If Action Reverse : Subsystem  TreatAsAtomicUnit=on
  Merge : Merge  Inputs=3
  OutputTorque = 0 : Constant  Value=0
  Product : Product  SaturateOnIntegerOverflow=on  InputSameDT=on  OutDataTypeStr=Inherit: Same as first input
  Product1 : Product  SaturateOnIntegerOverflow=on  InputSameDT=on  OutDataTypeStr=Inherit: Same as first input
  Transmission Gear ratios : Lookup  InputValues=p.tr_in  Table=p.tr_out  SaturateOnIntegerOverflow=on
  tTransmissionOut_[Nm] : Outport  InitialOutput=0
  nTransmissionIn_[rpm] : Outport  Port=2  InitialOutput=0
  wires:
  GearNr_[-]/1 -> Transmission Gear ratios/1, If/1
  If/3 -> If Action Normal/Action
  If/2 -> If Action Reverse/Action
  If Action Normal/1(Out1) -> Merge/3
  If Action Reverse/1(Out1) -> Merge/2
  If/1 -> If Action Neutral/Action
  If Action Neutral/1(Out1) -> Merge/1
  Product1/1 -> Ensure positive TransmissionRPM/1
  Merge/1 -> tTransmissionOut_[Nm]/1
  Product/1 -> If Action Reverse/1(In1), If Action Normal/1(In1)
  OutputTorque = 0/1 -> If Action Neutral/1(In1)
  Transmission Gear ratios/1 -> Product/2, Product1/1
  nTransmissionOut_[rpm]/1 -> Product1/2
  tTransmissionIn_[Nm]/1 -> Product/1
  Ensure positive TransmissionRPM/1 -> nTransmissionIn_[rpm]/1

== system Experiment_2_cs/Audi_A8_1/ENABLED/PPS Model/Actuation/Braking Lights ==
  note: === Braking lights block ===
      |
      |    - according to brake pressure, lights up braking lights of the actor,
      |    - the signal is a 3x1 vector:
      |      = first        value - left braking light,
      |      = second value - middle braking light,
      |      = third       value - right braking light.
  switcher : Inport
  Add : Sum
  Constant : Constant
  Constant1 : Constant  Value=0
  Mux : Mux  Inputs=3
  Pulse Generator : DiscretePulseGenerator  PulseType=Time based  Period=0.6  PulseWidth=50  PhaseDelay=0.3
  Rate Transition3 : RateTransition  Integrity=off  Deterministic=off  OutPortSampleTime=[0,0]
  Switch : Switch  Criteria=u2 > Threshold
  Switch1 : Switch  Criteria=u2 > Threshold
  Switch2 : Switch  Criteria=u2 > Threshold
  Unary Minus : UnaryMinus
  BrakeLights (3x1) : Outport
  wires:
  Mux/1 -> BrakeLights (3x1)/1
  switcher/1 -> Switch/2, Switch1/2, Switch2/2
  Constant/1 -> Switch/1, Add/2
  Switch/1 -> Switch1/3, Switch2/3, Mux/2
  Constant1/1 -> Switch/3
  Switch2/1 -> Mux/1
  Switch1/1 -> Mux/3
  Pulse Generator/1 -> Rate Transition3/1
  Add/1 -> Switch1/1
  Unary Minus/1 -> Add/1
  Rate Transition3/1 -> Unary Minus/1, Switch2/1

== system Experiment_2_cs/Audi_A8_1/ENABLED/PPS Model/Actuation/If Action Subsystem ==
  Action Port : ActionPort  ActionType=then
  Constant1 : Constant  SampleTime=[0,0]
  Data Store Write : DataStoreWrite  DialogController=Simulink.DDGSource  DataStoreName=full_brake
  wires:
  Constant1/1 -> Data Store Write/1

== system Experiment_2_cs/Audi_A8_1/ENABLED/PPS Model/PPS EGO State Display/Display function ==
  V [km/h] : Inport
  RPM : Inport  Port=2
  Brake Pressure : Inport  Port=3
  Detection flag : Inport  Port=4
  Warning Flag : Inport  Port=5
  Braking flag : Inport  Port=6
  Pet det flag : Inport  Port=7
  TTC : Inport  Port=8
  Enable : EnablePort
  Brake Pressure [bar]2 : Gain  Gain=100/MaxBrakePressure
  EGO Vehicle state display : M-S-Function  FunctionName=msfcn_PPS_PlotSpeed  Parameters=DisplayFreq DisplaySwitch
  Rounding Function2 : Rounding  Operator=round
  Rounding Function3 : Rounding  Operator=round
  wires:
  Brake Pressure [bar]2/1 -> Rounding Function3/1
  Rounding Function3/1 -> EGO Vehicle state display/3
  Rounding Function2/1 -> EGO Vehicle state display/2
  V [km/h]/1 -> EGO Vehicle state display/1
  Detection flag/1 -> EGO Vehicle state display/4
  Warning Flag/1 -> EGO Vehicle state display/5
  Braking flag/1 -> EGO Vehicle state display/6
  Pet det flag/1 -> EGO Vehicle state display/7
  TTC/1 -> EGO Vehicle state display/8
  RPM/1 -> Rounding Function2/1
  Brake Pressure/1 -> Brake Pressure [bar]2/1

== system Experiment_2_cs/Audi_A8_1/ENABLED/PPS Model/PPS EGO State Display/Plots ==
  V : Inport
  Ax : Inport  Port=2  SampleTime=[0,0]
  det : Inport  Port=3
  warn : Inport  Port=4
  brake : Inport  Port=5
  ped : Inport  Port=6
  ttc : Inport  Port=7
  Coll : Inport  Port=8
  Constant : Constant  Value=0
  Data Type Conversion4 : DataTypeConversion  OutDataTypeStr=double
  Mux : Mux
  Mux1 : Mux
  Rate Transition5 : RateTransition  Integrity=off  OutPortSampleTime=1/DisplayFreq
  Switch1 : Switch  Threshold=4
  To Workspace : ToWorkspace  VariableName=VRU_EGO_State_Flag06  SampleTime=-1
      settings: MaxDataPoints=1
  To Workspace1 : ToWorkspace  VariableName=VRU_EGO_State_BrakeVel  SampleTime=1/Mainfreq
      settings: MaxDataPoints=1
  To Workspace2 : ToWorkspace  VariableName=VRU_simout  SaveFormat=Structure With Time  SampleTime=0.04
  wires:
  Mux/1 -> To Workspace2/1
  Mux1/1 -> Data Type Conversion4/1
  Data Type Conversion4/1 -> Mux/3
  Ax/1 -> Rate Transition5/1
  Rate Transition5/1 -> Mux/2
  Switch1/1 -> Mux/4
  Constant/1 -> Switch1/1
  V/1 -> Mux/1
  det/1 -> Mux1/1
  warn/1 -> Mux1/2
  brake/1 -> Mux1/3, To Workspace/1
  ped/1 -> Mux1/4
  ttc/1 -> Switch1/2, Switch1/3
  Coll/1 -> To Workspace1/1

== system Experiment_2_cs/Audi_A8_1/ENABLED/PPS Model/PPS_Radar/Radar ==
  Range : Inport
  Theta : Inport  Port=2
  All flags : Inport  Port=3
  Flag 0.6 : Inport  Port=4
  Enable : EnablePort
  DISPLAY1 : M-S-Function  FunctionName=msfcn_PPS_radar_graph  Parameters=RadarFreq TISdet RadarSwitch TISMaxRange TISMaxTheta*pi/180
  Degrees to Radians : simulink_extras/Transformations/Degrees to Radians
  wires:
  Range/1 -> DISPLAY1/1
  Theta/1 -> Degrees to Radians/1
  All flags/1 -> DISPLAY1/3
  Flag 0.6/1 -> DISPLAY1/4
  Degrees to Radians/1 -> DISPLAY1/2

== system Experiment_2_cs/Audi_A8_1/ENABLED/PPS Model/Pedestrian detection/Blob Analysis ==
  orig_image : Inport
  proc_imag : Inport  Port=2
  posObj_subim : Inport  Port=3
  im_x : Inport  Port=4
  im_y : Inport  Port=5
  liminf_x : Inport  Port=6
  liminf_y : Inport  Port=7
  Blob Analysis1 : visionstatistics/Blob Analysis  Tag=vipblks_row_conv  area=off  centroid=on  bBox=on  majorAxis=on  minorAxis=on  angle=on  eccentricity=on  equivDiameterSq=off  extent=off  perimeter=off  maxBlobs=100  warnIfNumBlobsExceeded=on  isCount=off  useMinArea=on  minArea=50  useMaxArea=on  maxArea=150000  excludeBorderBlob=off  outDT=single  isOutVarDim=off  isFill=on  fillValues=-1  conn=4  isLabel=on  outputMode=Binary point scaling  outputWordLength=32  outputFracLength=16  firstCoeffMode=Binary point scaling  firstCoeffWordLength=16  firstCoeffFracLength=14  secondCoeffMode=Binary point scaling  secondCoeffWordLength=32  secondCoeffFracLength=16  accumMode=Binary point scaling  accumWordLength=32  accumFracLength=0  prodOutputMode=Binary point scaling  prodOutputWordLength=32  prodOutputFracLength=16  roundingMode=Floor  overflowMode=off
  Constant : Constant  Value=180/pi  VectorParams1D=off
  Data Type Conversion1 : DataTypeConversion  OutDataTypeStr=uint8
  Data Type Conversion2 : DataTypeConversion  OutDataTypeStr=uint8
  Data Type Conversion3 : DataTypeConversion  OutDataTypeStr=uint8
  Data Type Conversion4 : DataTypeConversion  OutDataTypeStr=boolean
  Draw Shapes1 : visiontextngfix/Draw Shapes  shape=Rectangles  fill=off  lineWidth=1  fillClrSource=Specify via dialog  display=White  intensity=200  color=[200 255 100]  opacity=0.6  viewport=Entire image  antialiasing=off  inType=Obsolete  imagePorts=One multidimensional signal  prodOutputMode=Binary point scaling  prodOutputWordLength=32  prodOutputFracLength=14  memoryMode=Specify word length  memoryWordLength=16  memoryFracLength=15  roundingMode=Floor  overflowMode=off
  Embedded MATLAB Function1 : MATLAB Function  TreatAsAtomicUnit=on
  Embedded MATLAB Function2 : MATLAB Function  TreatAsAtomicUnit=on
  Insert Text1 : visiontextngfix/Insert Text  inputType=Obsolete  theText='%02d'  getTextLocFrom=Input port  textLoc=[1 1]  getTextColorFrom=Input port  textColor=[0 0 0]  getTextIntensityFrom=Specify via dialog  textIntensity=0  getTextOpacityFrom=Specify via dialog  textOpacity=1.0  dummyVar2=0  dummyVar3=0  dummyVar4=0  imagePorts=One multidimensional signal  isInputTransposed=off  fontFace=LucidaSansRegular  dummyVar1=0  blockFontSize=12  antiAliased=on
  MATLAB Function : MATLAB Function  TreatAsAtomicUnit=on
  PEDES1 : MATLAB Function  TreatAsAtomicUnit=on
  PEDES2 : MATLAB Function  TreatAsAtomicUnit=on
  PEDES3 : MATLAB Function  TreatAsAtomicUnit=on
  PEDES4 : MATLAB Function  TreatAsAtomicUnit=on
  Product : Product  RndMeth=Zero
  Transpose : Subsystem
  Transpose1 : Subsystem
  Transpose2 : Subsystem
  Transpose3 : Subsystem
  Transpose4 : Subsystem
  Transpose5 : Subsystem
  Transpose6 : Subsystem
  Transpose7 : Subsystem
  BlobIm : Outport
  posObj_subim1 : Outport  Port=2
  Centroid_subim : Outport  Port=3
  BBox : Outport  Port=4
  wires:
  Blob Analysis1/4 -> Transpose5/1(U)
  Constant/1 -> Product/2
  Embedded MATLAB Function2/1(r_label) -> Data Type Conversion1/1
  Embedded MATLAB Function2/2(color) -> Data Type Conversion3/1
  Draw Shapes1/1 -> Data Type Conversion2/1
  Data Type Conversion1/1 -> Insert Text1/2
  Data Type Conversion2/1 -> Insert Text1/1
  Data Type Conversion3/1 -> Insert Text1/3
  Blob Analysis1/1 -> Transpose/1(U)
  Blob Analysis1/2 -> Transpose1/1(U)
  Blob Analysis1/3 -> Transpose2/1(U)
  Blob Analysis1/5 -> Transpose7/1(U)
  Product/1 -> Embedded MATLAB Function1/5(orientation)
  Blob Analysis1/7 -> Embedded MATLAB Function1/7(label)
  Embedded MATLAB Function1/3(label_out) -> Embedded MATLAB Function2/2(label)
  Embedded MATLAB Function1/2(bboxout) -> Embedded MATLAB Function2/1(nbboxout), BBox/1, MATLAB Function/1(u), PEDES4/1(pts)
  Embedded MATLAB Function1/1(centout) -> Centroid_subim/1
  Insert Text1/1 -> BlobIm/1
  proc_imag/1 -> Data Type Conversion4/1
  im_x/1 -> Embedded MATLAB Function1/8(im_x)
  orig_image/1 -> Draw Shapes1/1
  im_y/1 -> Embedded MATLAB Function1/9(im_y)
  liminf_x/1 -> Embedded MATLAB Function1/11(liminf_x)
  liminf_y/1 -> Embedded MATLAB Function1/12(liminf_y)
  posObj_subim/1 -> Embedded MATLAB Function1/10(posObj_subim)
  Embedded MATLAB Function1/4(posObj_im) -> posObj_subim1/1
  Data Type Conversion4/1 -> Blob Analysis1/1
  Blob Analysis1/6 -> Transpose6/1(U)
  PEDES1/1(inpoints) -> Insert Text1/4
  Transpose/1(Y) -> PEDES3/1(pts)
  Transpose1/1(Y) -> PEDES2/1(pts)
  Transpose3/1(Y) -> Draw Shapes1/2
  PEDES2/1(inpoints) -> Embedded MATLAB Function1/2(bbox)
  PEDES3/1(inpoints) -> Embedded MATLAB Function1/1(centroid)
  Transpose4/1(Y) -> PEDES1/1(pts)
  PEDES4/1(inpoints) -> Transpose3/1(U)
  Transpose7/1(Y) -> Product/1
  Transpose6/1(Y) -> Embedded MATLAB Function1/6(eccentricity)
  Transpose5/1(Y) -> Embedded MATLAB Function1/4(minoraxis)
  Transpose2/1(Y) -> Embedded MATLAB Function1/3(majoraxis)
  MATLAB Function/1(y) -> Transpose4/1(U)

== system Experiment_2_cs/Audi_A8_1/ENABLED/PPS Model/Pedestrian detection/Image processing ==
  Image : Inport
  Closing : visionmorphops/Closing  nhoodsrc=Specify via dialog  strel=strel('disk', 4)
  Edge Detection : visionanalysis/Edge Detection  method=Canny  outputType=Binary image  userDefinedThreshold=off  thresholdSource=Specify via dialog  threshold=1  thresholdTuning=3  edgeThinning=off  threshold_canny=[0.25 0.60]  autoPercent=93  sigma=1  prodOutputMode=Binary point scaling  prodOutputWordLength=32  prodOutputFracLength=8  roundingMode=Floor  overflowMode=off
  Embedded MATLAB Function : MATLAB Function  TreatAsAtomicUnit=on
  Image Data Type Conversion1 : visionconversions/Image Data Type Conversion  outDT=single  isSigned=on  wordLen=16  numFracBits=0
  ProcIm : Outport
  wires:
  Closing/1 -> Embedded MATLAB Function/1(image)
  Embedded MATLAB Function/1(im) -> ProcIm/1
  Image/1 -> Image Data Type Conversion1/1
  Edge Detection/1 -> Closing/1
  Image Data Type Conversion1/1 -> Edge Detection/1

== system Experiment_2_cs/Audi_A8_1/ENABLED/PPS Model/Pedestrian detection/Transpose ==
  U : Inport
  Data Type Conversion : DataTypeConversion
  Data Type Conversion1 : DataTypeConversion
  Interpreted MATLAB Function : MATLABFcn  MATLABFcn=transpose  Output1D=off
  Y : Outport
  wires:
  Data Type Conversion1/1 -> Y/1
  Interpreted MATLAB Function/1 -> Data Type Conversion1/1
  Data Type Conversion/1 -> Interpreted MATLAB Function/1
  U/1 -> Data Type Conversion/1
